simulink model "fcs_lab_07_model_01"  (R2014b)
settings: Solver=ode45  StartTime=0.0  StopTime=10.0  RelTol=1e-3
values from neighbouring files (symbols this model uses):
  b = 1    [fcs_lab_07_test.m]
  J = 0.01    [fcs_lab_07_test.m]
  K = 0.01    [fcs_lab_07_test.m]
  L = 0.5    [fcs_lab_07_test.m]
  R = 1    [fcs_lab_07_test.m]
settings Model: Creator=Mashkoor Ahmed  LastModifiedBy=Mashkoor Ahmed

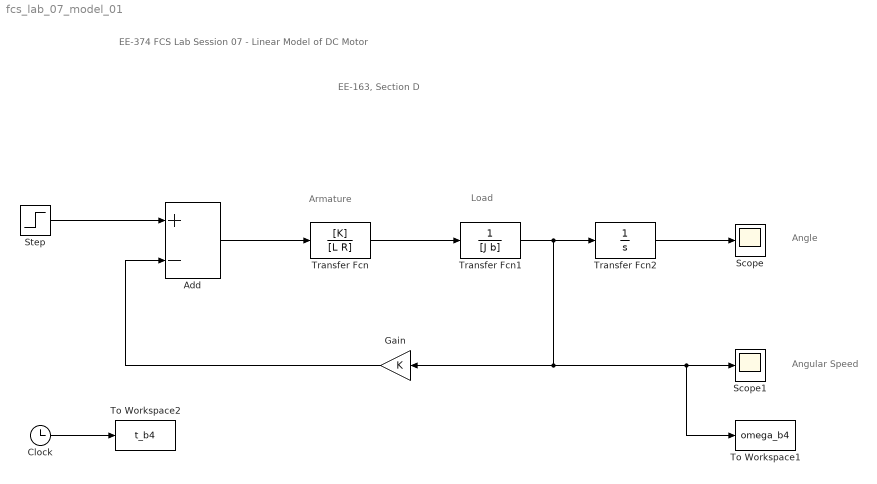
== system fcs_lab_07_model_01 ==
  note: EE-163, Section D
  note: EE-374 FCS Lab Session 07 - Linear Model of DC Motor
  note: Load
  note: Armature
  note: Angle
  note: Angular Speed
  Add : Sum  Inputs=+-
  Clock : Clock
  Gain : Gain  Gain=K
  Scope : Scope
  Scope1 : Scope
  Step : Step  Time=0  SampleTime=0
  To Workspace1 : ToWorkspace  VariableName=omega_b4  SampleTime=-1
  To Workspace2 : ToWorkspace  VariableName=t_b4  SampleTime=-1
  Transfer Fcn : TransferFcn  Numerator=[K]  Denominator=[L R]
  Transfer Fcn1 : TransferFcn  Denominator=[J b]
  Transfer Fcn2 : TransferFcn  Denominator=[1 0]
  wires:
  Step/1 -> Add/1
  Transfer Fcn/1 -> Transfer Fcn1/1
  Add/1 -> Transfer Fcn/1
  Transfer Fcn1/1 -> Gain/1, To Workspace1/1, Scope1/1, Transfer Fcn2/1
  Transfer Fcn2/1 -> Scope/1
  Gain/1 -> Add/2
  Clock/1 -> To Workspace2/1
